simulink model "P_d"  (Simulink 8.6)
settings: Solver=VariableStepAuto  StartTime=0.0  StopTime=20  RelTol=1e-3
values from neighbouring files (symbols this model uses):
  Dm = 0.2    [Parameters.m]
  Ds = 0.1    [Parameters.m]
  K = ceil(max(K1,K2))    [Gains.m]
  Lm1 = 0.5    [Parameters.m]
  Lm2 = 0.5    [Parameters.m]
  Ls1 = 0.5    [Parameters.m]
  Ls2 = 0.5    [Parameters.m]
  Mm1 = 1    [Parameters.m]
  Mm2 = 1    [Parameters.m]
  Ms1 = 2    [Parameters.m]
  Ms2 = 2    [Parameters.m]
  P = 10    [Parameters.m]
  q0 = [0;0]    [Parameters.m]
  v0 = [0;0;0]    [Initiation.m]    (also in Parameters.m = [0;0])
settings Model: Creator=TOSHIBA  LastModifiedBy=TOSHIBA
settings DataIOCC: SaveFormat=Dataset  SignalLoggingSaveFormat=Dataset
settings OptimizationCC: ExpressionDepthLimit=128
settings DebuggingCC: UnderspecifiedInitializationDetection=Simplified  MergeDetectMultiDrivingBlocksExec=error  SolverPrmCheckMsg=none  FcnCallInpInsideContextMsg=EnableAllAsError  StateNameClashWarn=none
settings HardwareCC: ProdBitPerPointer=64  ProdLargestAtomicFloat=Float  ProdIntDivRoundTo=Zero  ProdEndianess=LittleEndian  ProdWordSize=64  ProdHWDeviceType=Intel->x86-64 (Windows64)
settings GRTTargetCC: GeneratePreprocessorConditionals=Use local settings  CombineOutputUpdateFcns=on  GRTInterface=off
settings ConfigComp: CovModelRefEnable=off

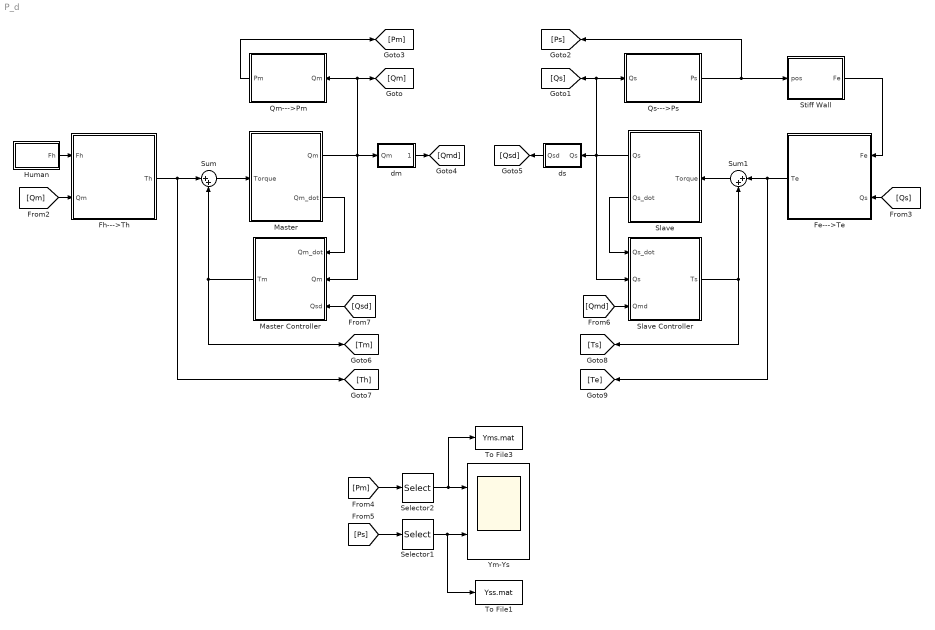
== system P_d ==
  Fe--->Te : Subsystem
  Fh--->Th : Subsystem
  Human : Subsystem
  Master : Subsystem
  Master Controller : Subsystem
  Qm--->Pm : Subsystem
  Qs--->Ps : Subsystem
  Selector1 : Selector  InputPortWidth=2  IndexOptions=Index vector (dialog)  Indices=[2]  OutputSizes=1
  Selector2 : Selector  InputPortWidth=2  IndexOptions=Index vector (dialog)  Indices=[2]  OutputSizes=1
  Slave : Subsystem
  Slave Controller : Subsystem
  Stiff Wall : MATLAB Function  TreatAsAtomicUnit=on
  Sum : Sum  Inputs=|++
  Sum1 : Sum  Inputs=|++
  To File1 : ToFile  Filename=Yss.mat  MatrixName=Yss  SaveFormat=Timeseries
  To File3 : ToFile  Filename=Yms.mat  MatrixName=Yms  SaveFormat=Timeseries
  Ym-Ys : Scope  NumInputPorts=2
  dm : Subsystem
  ds : Subsystem
  wires:
  Qs--->Ps/1(Ps) -> [Ps], Stiff Wall/1(pos)
  Stiff Wall/1(Fe) -> Fe--->Te/1(Fe)
  Fe--->Te/1(Te) -> Sum1/1, [Te]
  Sum1/1 -> Slave/1(Torque)
  Sum/1 -> Master/1(Torque)
  Fh--->Th/1(Th) -> [Th], Sum/1
  Master/2(Qm_dot) -> Master Controller/1(Qm_dot)
  Master Controller/1(Tm) -> Sum/2, [Tm]
  Slave/2(Qs_dot) -> Slave Controller/1(Qs_dot)
  Slave Controller/1(Ts) -> [Ts], Sum1/2
  [Qs] -> Fe--->Te/2(Qs)
  Master/1(Qm) -> dm/1(Qm), Qm--->Pm/1(Qm), [Qm], Master Controller/2(Qm)
  Slave/1(Qs) -> Slave Controller/2(Qs), ds/1(Qs), [Qs], Qs--->Ps/1(Qs)
  [Qm] -> Fh--->Th/2(Qm)
  Human/1(Fh) -> Fh--->Th/1(Fh)
  Qm--->Pm/1(Pm) -> [Pm]
  [Pm] -> Selector2/1
  Selector2/1 -> To File3/1, Ym-Ys/1
  [Qmd] -> Slave Controller/3(Qmd)
  dm/1(Qmd) -> [Qmd]
  ds/1(Qsd) -> [Qsd]
  [Qsd] -> Master Controller/3(Qsd)
  [Ps] -> Selector1/1
  Selector1/1 -> To File1/1, Ym-Ys/2

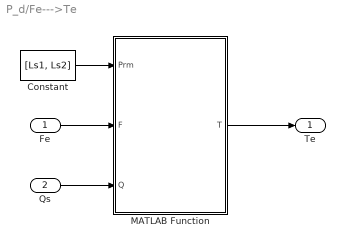
== system P_d/Fe--->Te ==
  Fe : Inport
  Qs : Inport  Port=2
  Constant : Constant  Value=[Ls1, Ls2]
  MATLAB Function : MATLAB Function  TreatAsAtomicUnit=on
  Te : Outport
  wires:
  Qs/1 -> MATLAB Function/3(Q)
  Fe/1 -> MATLAB Function/2(F)
  MATLAB Function/1(T) -> Te/1
  Constant/1 -> MATLAB Function/1(Prm)

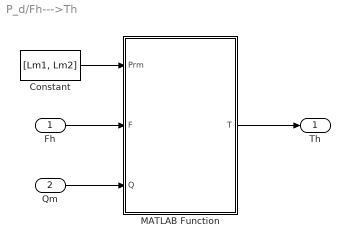
== system P_d/Fh--->Th ==
  Fh : Inport
  Qm : Inport  Port=2
  Constant : Constant  Value=[Lm1, Lm2]
  MATLAB Function : MATLAB Function  TreatAsAtomicUnit=on
  Th : Outport
  wires:
  Fh/1 -> MATLAB Function/2(F)
  MATLAB Function/1(T) -> Th/1
  Qm/1 -> MATLAB Function/3(Q)
  Constant/1 -> MATLAB Function/1(Prm)

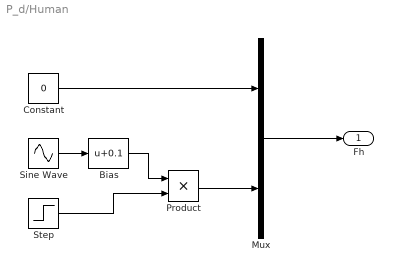
== system P_d/Human ==
  Bias : Bias  Bias=0.1
  Constant : Constant  Value=0
  Mux : Mux  Inputs=2
  Product : Product
  Sine Wave : Sin  Amplitude=0.4  Frequency=pi/5  SampleTime=0
  Step : Step  Time=100  Before=1  After=0  SampleTime=0
  Fh : Outport
  wires:
  Mux/1 -> Fh/1
  Constant/1 -> Mux/1
  Step/1 -> Product/2
  Bias/1 -> Product/1
  Product/1 -> Mux/2
  Sine Wave/1 -> Bias/1

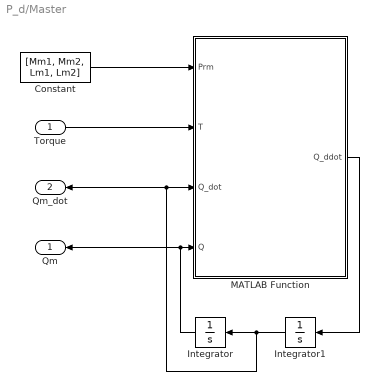
== system P_d/Master ==
  Torque : Inport
  Constant : Constant  Value=[Mm1, Mm2, Lm1, Lm2]
  Integrator : Integrator  InitialCondition=q0
  Integrator1 : Integrator  InitialCondition=v0
  MATLAB Function : MATLAB Function  TreatAsAtomicUnit=on
  Qm : Outport
  Qm_dot : Outport  Port=2
  wires:
  Torque/1 -> MATLAB Function/2(T)
  Constant/1 -> MATLAB Function/1(Prm)
  MATLAB Function/1(Q_ddot) -> Integrator1/1
  Integrator1/1 -> Qm_dot/1, MATLAB Function/3(Q_dot), Integrator/1
  Integrator/1 -> Qm/1, MATLAB Function/4(Q)

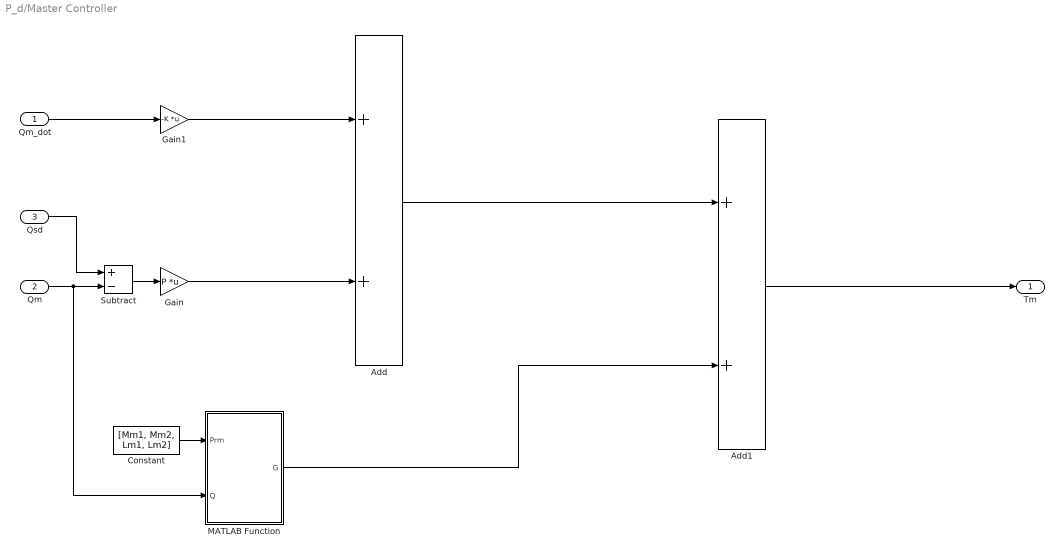
== system P_d/Master Controller ==
  Qm_dot : Inport
  Qm : Inport  Port=2
  Qsd : Inport  Port=3
  Add : Sum
  Add1 : Sum
  Constant : Constant  Value=[Mm1, Mm2, Lm1, Lm2]
  Gain : Gain  Gain=P  Multiplication=Matrix(K*u) (u vector)
  Gain1 : Gain  Gain=-K  Multiplication=Matrix(K*u) (u vector)
  MATLAB Function : MATLAB Function  TreatAsAtomicUnit=on
  Subtract : Sum  Inputs=+-
  Tm : Outport
  wires:
  Qm_dot/1 -> Gain1/1
  Subtract/1 -> Gain/1
  Gain/1 -> Add/2
  Gain1/1 -> Add/1
  Constant/1 -> MATLAB Function/1(Prm)
  Qm/1 -> Subtract/2, MATLAB Function/2(Q)
  Qsd/1 -> Subtract/1
  MATLAB Function/1(G) -> Add1/2
  Add1/1 -> Tm/1
  Add/1 -> Add1/1

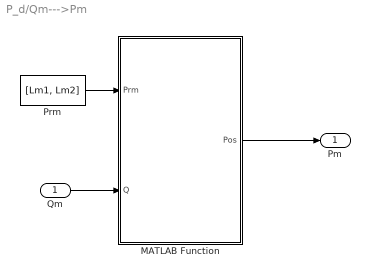
== system P_d/Qm--->Pm ==
  Qm : Inport
  MATLAB Function : MATLAB Function  TreatAsAtomicUnit=on
  Prm : Constant  Value=[Lm1, Lm2]
  Pm : Outport
  wires:
  MATLAB Function/1(Pos) -> Pm/1
  Qm/1 -> MATLAB Function/2(Q)
  Prm/1 -> MATLAB Function/1(Prm)

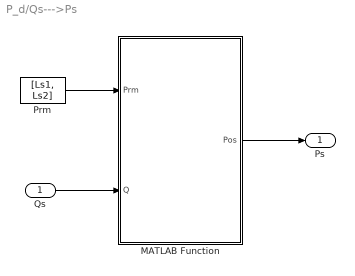
== system P_d/Qs--->Ps ==
  Qs : Inport
  MATLAB Function : MATLAB Function  TreatAsAtomicUnit=on
  Prm : Constant  Value=[Ls1, Ls2]
  Ps : Outport
  wires:
  Qs/1 -> MATLAB Function/2(Q)
  MATLAB Function/1(Pos) -> Ps/1
  Prm/1 -> MATLAB Function/1(Prm)

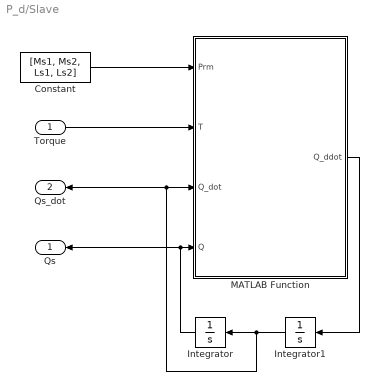
== system P_d/Slave ==
  Torque : Inport
  Constant : Constant  Value=[Ms1, Ms2, Ls1, Ls2]
  Integrator : Integrator  InitialCondition=q0
  Integrator1 : Integrator  InitialCondition=v0
  MATLAB Function : MATLAB Function  TreatAsAtomicUnit=on
  Qs : Outport
  Qs_dot : Outport  Port=2
  wires:
  Torque/1 -> MATLAB Function/2(T)
  Constant/1 -> MATLAB Function/1(Prm)
  MATLAB Function/1(Q_ddot) -> Integrator1/1
  Integrator1/1 -> Qs_dot/1, MATLAB Function/3(Q_dot), Integrator/1
  Integrator/1 -> Qs/1, MATLAB Function/4(Q)

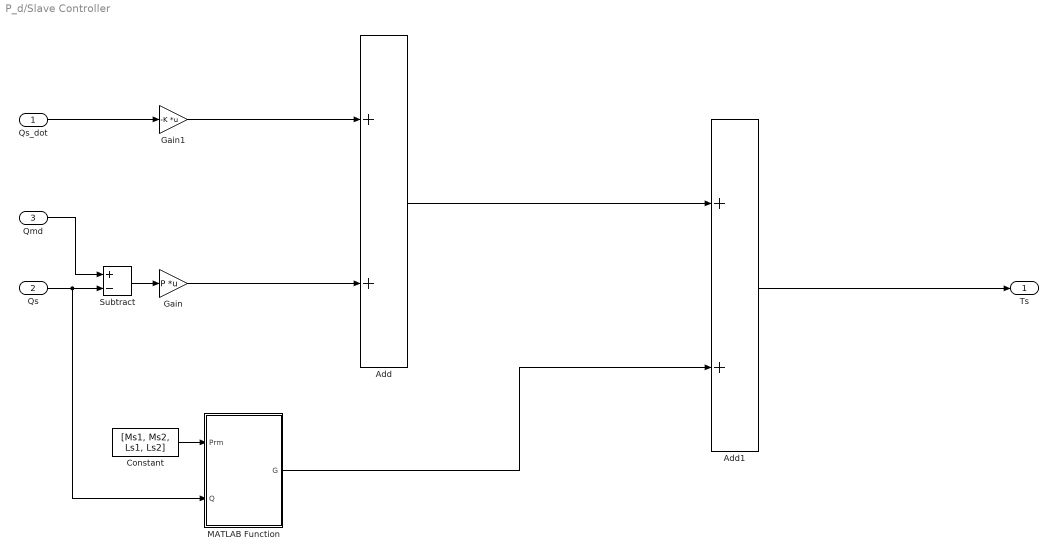
== system P_d/Slave Controller ==
  Qs_dot : Inport
  Qs : Inport  Port=2
  Qmd : Inport  Port=3
  Add : Sum
  Add1 : Sum
  Constant : Constant  Value=[Ms1, Ms2, Ls1, Ls2]
  Gain : Gain  Gain=P  Multiplication=Matrix(K*u) (u vector)
  Gain1 : Gain  Gain=-K  Multiplication=Matrix(K*u) (u vector)
  MATLAB Function : MATLAB Function  TreatAsAtomicUnit=on
  Subtract : Sum  Inputs=+-
  Ts : Outport
  wires:
  Qs_dot/1 -> Gain1/1
  Subtract/1 -> Gain/1
  Gain1/1 -> Add/1
  Constant/1 -> MATLAB Function/1(Prm)
  Qs/1 -> Subtract/2, MATLAB Function/2(Q)
  Qmd/1 -> Subtract/1
  MATLAB Function/1(G) -> Add1/2
  Add1/1 -> Ts/1
  Add/1 -> Add1/1
  Gain/1 -> Add/2

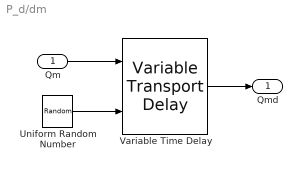
== system P_d/dm ==
  Qm : Inport
  Uniform Random Number : UniformRandomNumber  Minimum=0  Maximum=Dm  SampleTime=0.1
  Variable Time Delay : VariableTransportDelay  MaximumDelay=Dm
  Qmd : Outport
  wires:
  Qm/1 -> Variable Time Delay/1
  Uniform Random Number/1 -> Variable Time Delay/2
  Variable Time Delay/1 -> Qmd/1

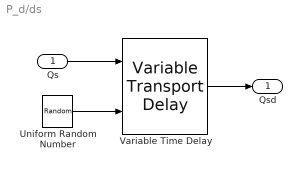
== system P_d/ds ==
  Qs : Inport
  Uniform Random Number : UniformRandomNumber  Minimum=0  Maximum=Ds  SampleTime=0.1
  Variable Time Delay : VariableTransportDelay  MaximumDelay=Ds
  Qsd : Outport
  wires:
  Uniform Random Number/1 -> Variable Time Delay/2
  Qs/1 -> Variable Time Delay/1
  Variable Time Delay/1 -> Qsd/1

== matlab function Master/MATLAB Function ==
  data: Prm input double; Q_ddot output double; T input double; Q_dot input double; Q input double
function Q_ddot  = RobotArm_2DOF(Prm, T, Q_dot, Q)
%#eml
g = 9.8;
m1 = Prm(1);
m2 = Prm(2);
l1 = Prm(3);
l2 = Prm(4);
q1 = Q(1);
q2 = Q(2);
q1_dot = Q_dot(1);
q2_dot = Q_dot(2);
M11 = m2*l2^2+(m1+m2)*l1^2+2*m2*l1*l2*cos(q2);
M12 = m2*l2^2+m2*l1*l2*cos(q2);
M21 = M12;
M22 = m2*l2^2;
M = [M11, M12; M21, M22];
C11 = -2*m2*l1*l2*sin(q2)*q2_dot;
C12 = -m2*l1*l2*sin(q2)*q2_dot;
C21 = m2*l1*l2*sin(q2)*q1_dot;
C22 = 0;
C = [C11, C12; C21, C22];
g1 = m2*g*l2*sin(q1+q2)+(m1+m2)*g*l1*sin(q1);
g2 = m2*g*l2*sin(q1+q2);
G = [g1; g2];
Q_ddot = M\(T-C*Q_dot-G);

== matlab function Stiff Wall ==
  data: pos input double; Fe output double
function Fe  = Envir(pos)
%#eml
kWall = 1000;
if pos(2)>=0.2
    Fe=[0; -(pos(2)-0.2)*kWall];
    if Fe(2)>0
        Fe = zeros(2,1);
    end
else
    Fe=zeros(2,1);
end

== matlab function Slave/MATLAB Function ==
  data: Prm input double; Q_ddot output double; T input double; Q_dot input double; Q input double
function Q_ddot  = RobotArm_2DOF(Prm, T, Q_dot, Q)
%#eml
g = 9.8;
m1 = Prm(1);
m2 = Prm(2);
l1 = Prm(3);
l2 = Prm(4);
q1 = Q(1);
q2 = Q(2);
q1_dot = Q_dot(1);
q2_dot = Q_dot(2);
M11 = m2*l2^2+(m1+m2)*l1^2+2*m2*l1*l2*cos(q2);
M12 = m2*l2^2+m2*l1*l2*cos(q2);
M21 = M12;
M22 = m2*l2^2;
M = [M11, M12; M21, M22];
C11 = -2*m2*l1*l2*sin(q2)*q2_dot;
C12 = -m2*l1*l2*sin(q2)*q2_dot;
C21 = m2*l1*l2*sin(q2)*q1_dot;
C22 = 0;
C = [C11, C12; C21, C22];
g1 = m2*g*l2*sin(q1+q2)+(m1+m2)*g*l1*sin(q1);
g2 = m2*g*l2*sin(q1+q2);
G = [g1; g2];
Q_ddot = M\(T-C*Q_dot-G);

== matlab function Qm--->Pm/MATLAB Function ==
  data: Prm input double; Pos output double; Q input double
function Pos = ForwardKinematics(Prm, Q)
%#eml
l1 = Prm(1);
l2 = Prm(2);
q1 = Q(1);
q2 = Q(2);
x = l1*cos(q1)+l2*cos(q1+q2);
y = l1*sin(q1)+l2*sin(q1+q2);
Pos = [x; y];

== matlab function Qs--->Ps/MATLAB Function ==
  data: Prm input double; Pos output double; Q input double
function Pos = ForwardKinematics(Prm, Q)
%#eml
l1 = Prm(1);
l2 = Prm(2);
q1 = Q(1);
q2 = Q(2);
x = l1*cos(q1)+l2*cos(q1+q2);
y = l1*sin(q1)+l2*sin(q1+q2);
Pos = [x; y];

== matlab function Fh--->Th/MATLAB Function ==
  data: Prm input double; T output double; F input double; Q input double
function T = Force_to_Torque(Prm, F, Q)
%#eml
l1 = Prm(1);
l2 = Prm(2);
q1 = Q(1);
q2 = Q(2);
J11 = -l1*sin(q1)-l2*sin(q1+q2);
J12 = -l2*sin(q1+q2);
J21 = l1*cos(q1)+l2*cos(q1+q2);
J22 = l2*cos(q1+q2);
J = [J11, J12; J21, J22];
T = J'*F;

== matlab function Fe--->Te/MATLAB Function ==
  data: Prm input double; T output double; F input double; Q input double
function T = Force_to_Torque(Prm, F, Q)
%#eml
l1 = Prm(1);
l2 = Prm(2);
q1 = Q(1);
q2 = Q(2);
J11 = -l1*sin(q1)-l2*sin(q1+q2);
J12 = -l2*sin(q1+q2);
J21 = l1*cos(q1)+l2*cos(q1+q2);
J22 = l2*cos(q1+q2);
J = [J11, J12; J21, J22];
T = J'*F;

== matlab function Master Controller/MATLAB Function ==
  data: Prm input double; G output double; Q input double
function G = Gravity(Prm, Q)

g = 9.8;
m1 = Prm(1);
m2 = Prm(2);
l1 = Prm(3);
l2 = Prm(4);
q1 = Q(1);
q2 = Q(2);

g1 = m2*g*l2*sin(q1+q2)+(m1+m2)*g*l1*sin(q1);
g2 = m2*g*l2*sin(q1+q2);
G = [g1; g2];

== matlab function Slave Controller/MATLAB Function ==
  data: Prm input double; G output double; Q input double
function G = Gravity(Prm, Q)

g = 9.8;
m1 = Prm(1);
m2 = Prm(2);
l1 = Prm(3);
l2 = Prm(4);
q1 = Q(1);
q2 = Q(2);

g1 = m2*g*l2*sin(q1+q2)+(m1+m2)*g*l1*sin(q1);
g2 = m2*g*l2*sin(q1+q2);
G = [g1; g2];
